simulink model "AltControlSimulink"  (R2017b)
settings: Solver=VariableStepAuto  StartTime=0.0  StopTime=7200  RelTol=1e-3  EnableMultiTasking=on
settings Model: Creator=alexismitchnick  LastModifiedBy=merigelb
settings SolverCC: SolverJacobianMethodControl=FullAnalytical  ZeroCrossControl=DisableAll
settings OptimizationCC: LifeSpan=inf
settings DebuggingCC: SFUnexpectedBacktrackingDiag=warning  SFNoUnconditionalDefaultTransitionDiag=warning  SFExecutionAtInitializationDiag=none
settings CodeAppCC: StateflowObjectComments=on
settings GRTTargetCC: TargetLangStandard=C89/C90 (ANSI)  GeneratePreprocessorConditionals=Disable all
settings ConfigComp: CovMetricSettings=dw  CovHtmlReporting=on  CovSaveCumulativeToWorkspaceVar=on  CovSaveSingleToWorkspaceVar=on  CovExternalEMLEnable=off

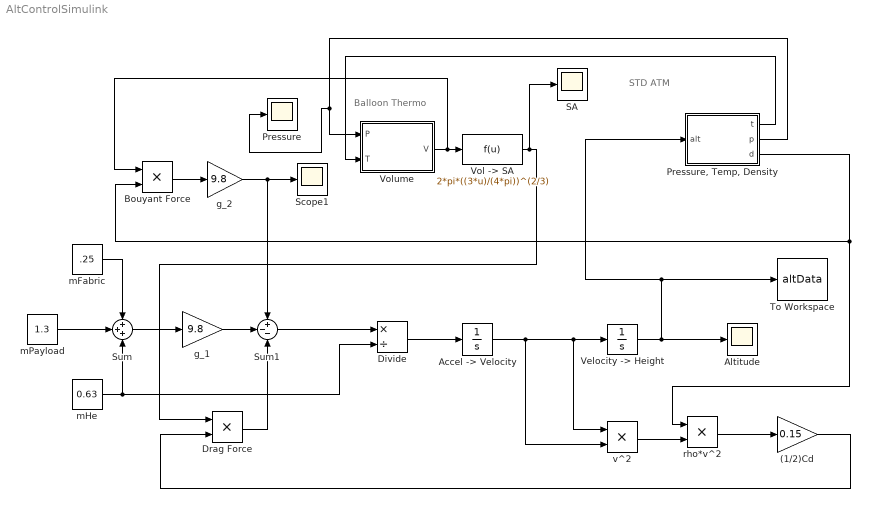
== system AltControlSimulink ==
  note: Balloon Thermo
  note: STD ATM
  (1/2)Cd : Gain  Gain=0.15
  "Accel -> Velocity" : Integrator
  "Altitude " : Scope
  Bouyant Force : Product
  Divide : Product  Inputs=*/
  Drag Force : Product
  Pressure : Scope
  "Pressure, Temp, Density" : MATLAB Function  TreatAsAtomicUnit=on
  SA : Scope
  Scope1 : Scope
  Sum : Sum  Inputs=+++
  Sum1 : Sum  Inputs=+--
  To Workspace : ToWorkspace  VariableName=altData  SampleTime=-1
      settings: Save2DSignal=2-D array (concatenate along first dimension)
  "Velocity -> Height" : Integrator
  "Vol -> SA" : Fcn  Expr=2*pi*((3*u)/(4*pi))^(2/3)
  Volume : MATLAB Function  TreatAsAtomicUnit=on
  "g_1 " : Gain  Gain=9.8
  g_2 : Gain  Gain=9.8
  mFabric : Constant  Value=.25
  mHe : Constant  Value=0.63
  mPayload : Constant  Value=1.3
  rho*v^2 : Product
  v^2 : Product
  wires:
  mFabric/1 -> Sum/1
  mPayload/1 -> Sum/2
  Sum/1 -> "g_1 "/1
  "g_1 "/1 -> Sum1/2
  mHe/1 -> Sum/3, Divide/2
  Sum1/1 -> Divide/1
  Divide/1 -> "Accel -> Velocity"/1
  "Accel -> Velocity"/1 -> "Velocity -> Height"/1, v^2/1, v^2/2
  Drag Force/1 -> Sum1/3
  "Pressure, Temp, Density"/3(d) -> rho*v^2/1, Bouyant Force/2
  "Vol -> SA"/1 -> SA/1, Drag Force/1
  v^2/1 -> rho*v^2/2
  rho*v^2/1 -> (1/2)Cd/1
  (1/2)Cd/1 -> Drag Force/2
  Bouyant Force/1 -> g_2/1
  "Velocity -> Height"/1 -> "Pressure, Temp, Density"/1(alt), To Workspace/1, "Altitude "/1
  Volume/1(V) -> Bouyant Force/1, "Vol -> SA"/1
  g_2/1 -> Scope1/1, Sum1/1
  "Pressure, Temp, Density"/2(p) -> Pressure/1, Volume/1(P)
  "Pressure, Temp, Density"/1(t) -> Volume/2(T)

== matlab function AltControlSimulink/Pressure, Temp, Density ==
  data: alt input; t output; p output; d output
function [t,p,d] = getTPD(alt)
    if alt <= 11000 %meters
        t = 15.04 - 0.00649*alt; %celcius
        p = 101.29 * ((t + 273.1)/288.08)^5.256; %kPa
    elseif (11000 < alt) && (alt <= 25000)
     
        t = -56.46;%celcius
        p = 22.65 * exp(1.73 - (0.000157*alt));
     else
         t = -131.21 + 0.00299*alt;
         p = 2.488 * ((t + 273.1)/216.6)^(-11.38);
    end
    d = p/(0.2869 * (t + 273.1));
end

== matlab function AltControlSimulink/Volume ==
  data: P input; V output; T input
function V = fcn(P,T)
mHe = 1.24;
R = 2.0769;
Pnew = P;
%Pnew = P/1000;
V = (mHe*R*(T+273))/Pnew;
